simulink library "Control_lib"  (Simulink 7.4)
settings: Solver=ode45  StartTime=0.0  StopTime=10.0  RelTol=1e-3
values from neighbouring files (symbols this model uses):
  f1 = (I_y-I_z)/I_x    [quadrocopter_param.m]
  f2 = rot.J_z/I_x    [quadrocopter_param.m]
  f3 = (I_z-I_x)/I_y    [quadrocopter_param.m]
  f4 = rot.J_z/I_y    [quadrocopter_param.m]
  f5 = (I_x-I_y)/I_z    [quadrocopter_param.m]
  g = 9.81    [quadrocopter_param.m]
  I_x = elec.I_x+bat.I_x+2*boom.I_1x+2*boom.I_1y+2*mot.I_1x+2*mot.I_1y+                             2*rot.I_1x+2*rot.I_1y    [quadrocopter_param.m]
  I_y = elec.I_y+bat.I_y+2*boom.I_1x+2*boom.I_1y+2*mot.I_1x+2*mot.I_1y+                             2*rot.I_1x+2*rot.I_1y    [quadrocopter_param.m]
  I_z = elec.I_z+bat.I_z+4*boom.I_1z+4*mot.I_1z+4*rot.I_1z    [quadrocopter_param.m]
  m = m*1.2    [quadrocopter_param.m]
  phi0 = 0    [quadrocopter_param.m]
  r_phi0 = 0    [quadrocopter_param.m]
  r_psi0 = 0    [quadrocopter_param.m]
  r_theta0 = 0    [quadrocopter_param.m]
  theta0 = 0    [quadrocopter_param.m]
  Ts = 0.005    [quadrocopter_param.m]
undefined symbols (not defined in the file or in its folder): boom, DiscIntNeverNeededParam
libraries: Copter_Library x10, simulink x5
settings Model: Creator=roczit00  LastModifiedBy=robert

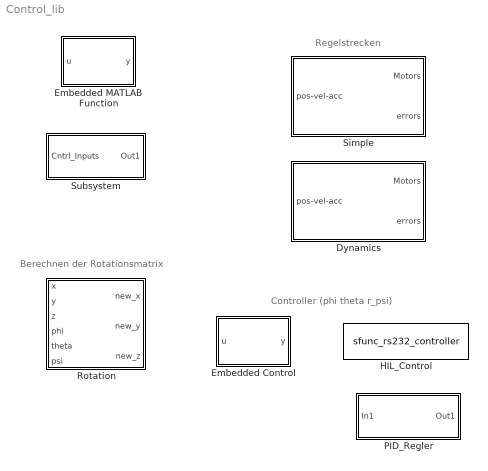
== system Control_lib ==
  note: Regelstrecken
  note: Berechnen der Rotationsmatrix
  note: Controller (phi theta r_psi)
  Dynamics : Subsystem
  Embedded Control : Stateflow chart
  Embedded MATLAB Function : Stateflow chart
  HIL_Control : S-Function  FunctionName=sfunc_rs232_controller  Parameters=Config  EnableBusSupport=off  mask{enabled=off}
      mask prompts: enabled "Enable this Block:"
      mask init:
      | Config.Enabled = enabled;
  PID_Regler : Subsystem
  Rotation : Subsystem
  Simple : Subsystem
  Subsystem : Subsystem  mask{G=9.81}
      mask prompts: G "Erdbeschleunigung [m/s²]:"
      mask init:
      | g = G;

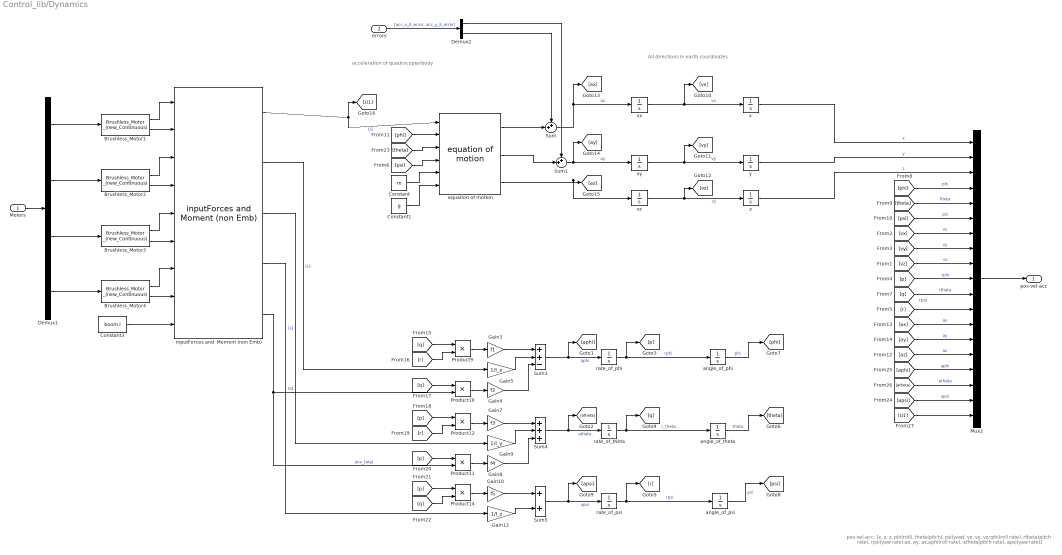
== system Control_lib/Dynamics ==
  note: rpsi
  note: pos-vel-acc: [x, y, z, phi(roll), theta(pitch), psi(yaw), vx, vy, vz,rphi(roll rate), rtheta(pitch rate), rpsi(yaw rate),ax, ay, az,aphi(roll rate), atheta(pitch rate), apsi(yaw rate)]
  note: All directions in earth coordinates
  note: acceleration of quadrocopterbody
  Motors : Inport  OutDataType=fixdt(1, 16)  OutScaling=2^0
  errors : Inport  Port=2  OutDataType=fixdt(1, 16)  OutScaling=2^0
  Brushless_Motor{1..4} (4 alike) : Copter_Library/Brushless_Motor _(new_Continuous)  SystemSampleTime=-1  M_error=0
  Constant : Constant  Value=m  OutDataType=fixdt(1, 16)  OutScaling=2^0
  Constant1 : Constant  Value=g  OutDataType=fixdt(1, 16)  OutScaling=2^0
  Constant3 : Constant  Value=boom.l  OutDataType=fixdt(1, 16)  OutScaling=2^0
  Demux1 : Demux
  Demux2 : Demux  Outputs=2
  Gain10 : Gain  Gain=f5  ParameterDataType=fixdt(1, 16)  ParameterScaling=2^0  OutDataType=fixdt(1, 16)  OutScaling=2^0
  Gain12 : Gain  Gain=1/I_z  ParameterDataType=fixdt(1, 16)  ParameterScaling=2^0  OutDataType=fixdt(1, 16)  OutScaling=2^0
  Gain3 : Gain  Gain=f1  ParameterDataType=fixdt(1, 16)  ParameterScaling=2^0  OutDataType=fixdt(1, 16)  OutScaling=2^0
  Gain4 : Gain  Gain=f2  ParameterDataType=fixdt(1, 16)  ParameterScaling=2^0  OutDataType=fixdt(1, 16)  OutScaling=2^0
  Gain5 : Gain  Gain=1/I_x  ParameterDataType=fixdt(1, 16)  ParameterScaling=2^0  OutDataType=fixdt(1, 16)  OutScaling=2^0
  Gain7 : Gain  Gain=f3  ParameterDataType=fixdt(1, 16)  ParameterScaling=2^0  OutDataType=fixdt(1, 16)  OutScaling=2^0
  Gain8 : Gain  Gain=f4  ParameterDataType=fixdt(1, 16)  ParameterScaling=2^0  OutDataType=fixdt(1, 16)  OutScaling=2^0
  Gain9 : Gain  Gain=1/I_y  ParameterDataType=fixdt(1, 16)  ParameterScaling=2^0  OutDataType=fixdt(1, 16)  OutScaling=2^0
  Mux2 : Mux  Inputs=19
  Product{9..12,14} (5 alike) : Product  OutDataType=fixdt(1, 16)  OutScaling=2^0  RndMeth=Zero
  Sum : Sum  Inputs=++|  OutDataType=fixdt(1, 16)  OutScaling=2^0
  Sum1 : Sum  Inputs=++|  OutDataType=fixdt(1, 16)  OutScaling=2^0
  Sum3 : Sum  Inputs=++-  OutDataType=fixdt(1, 16)  OutScaling=2^0
  Sum4 : Sum  Inputs=+++  OutDataType=fixdt(1, 16)  OutScaling=2^0
  Sum5 : Sum  OutDataType=fixdt(1, 16)  OutScaling=2^0
  angle_of_phi : Integrator  InitialCondition=phi0
  angle_of_psi : Integrator
  angle_of_theta : Integrator  InitialCondition=theta0
  equation of motion : Copter_Library/equation of motion  SystemSampleTime=-1
  inputForces and  Moment (non Emb) : Copter_Library/inputForces and  Moment (non Emb)  SystemSampleTime=-1
  rate_of_phi : Integrator  InitialCondition=r_phi0
  rate_of_psi : Integrator  InitialCondition=r_psi0
  rate_of_theta : Integrator  InitialCondition=r_theta0
  vx : Integrator
  vy : Integrator
  vz : Integrator
  x : Integrator
  y : Integrator
  z : Integrator
  pos-vel-acc : Outport  OutDataType=fixdt(1, 16)  OutScaling=2^0
  wires:
  [apsi] -> Mux2/18  "apsi"
  [atheta] -> Mux2/17  "atheta"
  [aphi] -> Mux2/16  "aphi"
  [az] -> Mux2/15  "az"
  [ay] -> Mux2/14  "ay"
  [ax] -> Mux2/13  "ax"
  [r] -> Mux2/12
  [q] -> Mux2/11  "rtheta"
  [p] -> Mux2/10  "rphi"
  [vz] -> Mux2/9  "vz"
  [vy] -> Mux2/8  "vy"
  [vx] -> Mux2/7  "vx"
  [psi] -> Mux2/6  "psi"
  [theta] -> Mux2/5  "theta"
  [phi] -> Mux2/4  "phi"
  z/1 -> Mux2/3  "z"
  Mux2/1 -> pos-vel-acc/1
  errors/1 -> Demux2/1  "[acc_x_E_error, acc_y_E_error]"
  Motors/1 -> Demux1/1
  Demux1/3 -> Brushless_Motor3/1
  Demux1/4 -> Brushless_Motor4/1
  Demux1/2 -> Brushless_Motor2/1
  Demux1/1 -> Brushless_Motor1/1
  vx/1 -> [vx], x/1  "vx"
  vy/1 -> [vy], y/1  "vy"
  vz/1 -> [vz], z/1  "vz"
  Constant3/1 -> inputForces and  Moment (non Emb)/9
  Sum5/1 -> [apsi], rate_of_psi/1  "apsi"
  inputForces and  Moment (non Emb)/4 -> Gain12/1  "U4"
  Gain12/1 -> Sum5/2
  Gain10/1 -> Sum5/1
  Product14/1 -> Gain10/1
  [q] -> Product14/2
  [p] -> Product14/1
  Sum4/1 -> [atheta], rate_of_theta/1  "atheta"
  inputForces and  Moment (non Emb)/3 -> Gain9/1  "U3"
  Gain8/1 -> Sum4/3
  Gain9/1 -> Sum4/2
  Product11/1 -> Gain8/1
  [p] -> Product11/1
  Gain7/1 -> Sum4/1
  Product12/1 -> Gain7/1
  [r] -> Product12/2
  [p] -> Product12/1
  Sum3/1 -> [aphi], rate_of_phi/1  "aphi"
  Gain4/1 -> Sum3/3
  Gain5/1 -> Sum3/2
  inputForces and  Moment (non Emb)/2 -> Gain5/1  "U2"
  Product10/1 -> Gain4/1
  [q] -> Product10/1
  Gain3/1 -> Sum3/1
  Product9/1 -> Gain3/1
  [r] -> Product9/2
  [q] -> Product9/1
  inputForces and  Moment (non Emb)/5 -> Product11/2, Product10/2  "anv_total"
  angle_of_phi/1 -> [phi]  "phi"
  angle_of_theta/1 -> [theta]  "theta"
  angle_of_psi/1 -> [psi]  "psi"
  rate_of_phi/1 -> [p], angle_of_phi/1  "rphi"
  rate_of_theta/1 -> angle_of_theta/1, [q]  "r_theta"
  rate_of_psi/1 -> angle_of_psi/1, [r]  "rpsi"
  Brushless_Motor1/1 -> inputForces and  Moment (non Emb)/1
  Brushless_Motor1/2 -> inputForces and  Moment (non Emb)/2
  Brushless_Motor2/1 -> inputForces and  Moment (non Emb)/3
  Brushless_Motor2/2 -> inputForces and  Moment (non Emb)/4
  Brushless_Motor3/1 -> inputForces and  Moment (non Emb)/5
  Brushless_Motor3/2 -> inputForces and  Moment (non Emb)/6
  Brushless_Motor4/1 -> inputForces and  Moment (non Emb)/7
  Brushless_Motor4/2 -> inputForces and  Moment (non Emb)/8
  x/1 -> Mux2/1  "x"
  y/1 -> Mux2/2  "y"
  Sum1/1 -> [ay], vy/1  "ay"
  Sum/1 -> [ax], vx/1  "ax"
  Demux2/2 -> Sum/1
  Demux2/1 -> Sum1/1
  equation of motion/3 -> [az], vz/1
  equation of motion/2 -> Sum1/2
  equation of motion/1 -> Sum/2
  inputForces and  Moment (non Emb)/1 -> equation of motion/1, [U1]  "U1"
  [phi] -> equation of motion/2
  [theta] -> equation of motion/3
  [psi] -> equation of motion/4
  Constant/1 -> equation of motion/5
  Constant1/1 -> equation of motion/6
  [U1] -> Mux2/19

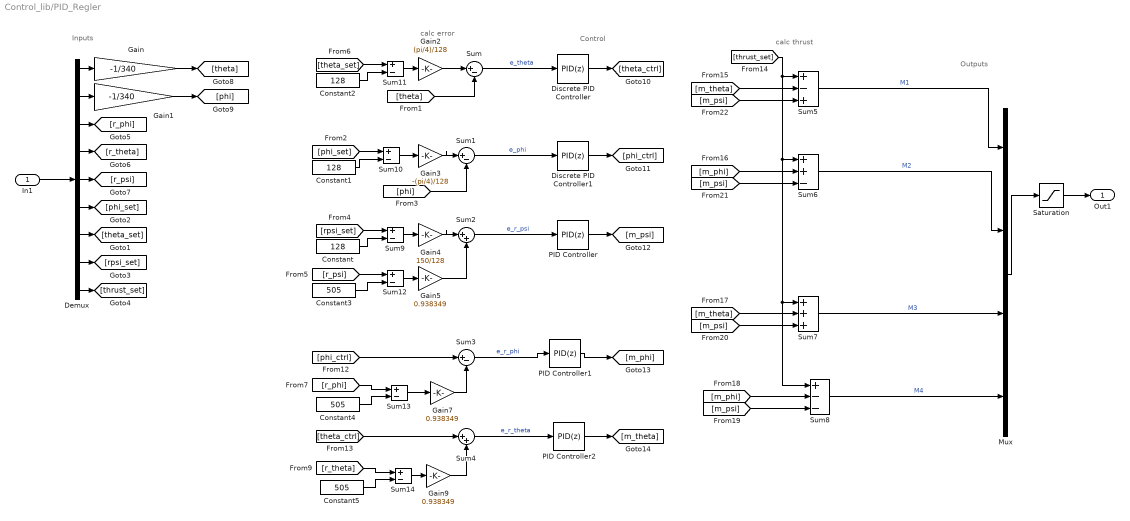
== system Control_lib/PID_Regler ==
  note: Inputs
  note: calc error
  note: Outputs
  note: Control
  note: calc thrust
  In1 : Inport  OutDataType=fixdt(1, 16)  OutScaling=2^0
  Constant : Constant  Value=128  OutDataType=fixdt(1, 16)  OutScaling=2^0
  Constant1 : Constant  Value=128  OutDataType=fixdt(1, 16)  OutScaling=2^0
  Constant2 : Constant  Value=128  OutDataType=fixdt(1, 16)  OutScaling=2^0
  Constant3 : Constant  Value=505  OutDataType=fixdt(1, 16)  OutScaling=2^0
  Constant4 : Constant  Value=505  OutDataType=fixdt(1, 16)  OutScaling=2^0
  Constant5 : Constant  Value=505  OutDataType=fixdt(1, 16)  OutScaling=2^0
  Demux : Demux  Outputs=9
  Discrete PID Controller : simulink/Continuous/PID Controller  DialogController=pidpack.PIDConfig.pidDDGCreate  DialogControllerArgs=DataTag0  SystemSampleTime=-1  Controller=PID  TimeDomain=Discrete-time  SampleTime=Ts  IntegratorMethod=Forward Euler  FilterMethod=Forward Euler  Form=Ideal  P=150  I=0.5  D=0  N=0  InitialConditionSource=internal  InitialConditionForIntegrator=0  InitialConditionForFilter=0  ExternalReset=none  ZeroCross=off  LimitOutput=off  UpperSaturationLimit=inf  LowerSaturationLimit=-inf  LinearizeAsGain=off  AntiWindupMode=none  Kb=1  TrackingMode=off  Kt=1  PParamMin=[]  PParamMax=[]  IParamMin=[]  IParamMax=[]  DParamMin=[]  DParamMax=[]  NParamMin=[]  NParamMax=[]  KbParamMin=[]  KbParamMax=[]  KtParamMin=[]  KtParamMax=[]  POutMin=[]  POutMax=[]  IOutMin=[]  IOutMax=[]  DOutMin=[]  DOutMax=[]  NOutMin=[]  NOutMax=[]  KbOutMin=[]  KbOutMax=[]  KtOutMin=[]  KtOutMax=[]  IntegratorOutMin=[]  IntegratorOutMax=[]  FilterOutMin=[]  FilterOutMax=[]  SumOutMin=[]  SumOutMax=[]  SumI1OutMin=[]  SumI1OutMax=[]  SumI2OutMin=[]  SumI2OutMax=[]  SumI3OutMin=[]  SumI3OutMax=[]  SumDOutMin=[]  SumDOutMax=[]  SaturationOutMin=[]  SaturationOutMax=[]  IntegratorContinuousStateAttributes=''  IntegratorStateMustResolveToSignalObject=off  IntegratorRTWStateStorageClass=Auto  FilterContinuousStateAttributes=''  FilterStateMustResolveToSignalObject=off  FilterRTWStateStorageClass=Auto
  Discrete PID Controller1 : simulink/Continuous/PID Controller  DialogController=pidpack.PIDConfig.pidDDGCreate  DialogControllerArgs=DataTag1  SystemSampleTime=-1  Controller=PID  TimeDomain=Discrete-time  SampleTime=Ts  IntegratorMethod=Forward Euler  FilterMethod=Forward Euler  Form=Ideal  P=150  I=0.5  D=0  N=0  InitialConditionSource=internal  InitialConditionForIntegrator=0  InitialConditionForFilter=0  ExternalReset=none  ZeroCross=off  LimitOutput=off  UpperSaturationLimit=inf  LowerSaturationLimit=-inf  LinearizeAsGain=off  AntiWindupMode=none  Kb=1  TrackingMode=off  Kt=1  PParamMin=[]  PParamMax=[]  IParamMin=[]  IParamMax=[]  DParamMin=[]  DParamMax=[]  NParamMin=[]  NParamMax=[]  KbParamMin=[]  KbParamMax=[]  KtParamMin=[]  KtParamMax=[]  POutMin=[]  POutMax=[]  IOutMin=[]  IOutMax=[]  DOutMin=[]  DOutMax=[]  NOutMin=[]  NOutMax=[]  KbOutMin=[]  KbOutMax=[]  KtOutMin=[]  KtOutMax=[]  IntegratorOutMin=[]  IntegratorOutMax=[]  FilterOutMin=[]  FilterOutMax=[]  SumOutMin=[]  SumOutMax=[]  SumI1OutMin=[]  SumI1OutMax=[]  SumI2OutMin=[]  SumI2OutMax=[]  SumI3OutMin=[]  SumI3OutMax=[]  SumDOutMin=[]  SumDOutMax=[]  SaturationOutMin=[]  SaturationOutMax=[]  IntegratorContinuousStateAttributes=''  IntegratorStateMustResolveToSignalObject=off  IntegratorRTWStateStorageClass=Auto  FilterContinuousStateAttributes=''  FilterStateMustResolveToSignalObject=off  FilterRTWStateStorageClass=Auto
  Gain : Gain  Gain=-1/340  ParameterDataType=fixdt(1, 16)  ParameterScaling=2^0  OutDataType=fixdt(1, 16)  OutScaling=2^0
  Gain1 : Gain  Gain=-1/340  ParameterDataType=fixdt(1, 16)  ParameterScaling=2^0  OutDataType=fixdt(1, 16)  OutScaling=2^0
  Gain2 : Gain  Gain=(pi/4)/128  ParameterDataType=fixdt(1, 16)  ParameterScaling=2^0  OutDataType=fixdt(1, 16)  OutScaling=2^0
  Gain3 : Gain  Gain=-(pi/4)/128  ParameterDataType=fixdt(1, 16)  ParameterScaling=2^0  OutDataType=fixdt(1, 16)  OutScaling=2^0
  Gain4 : Gain  Gain=150/128  ParameterDataType=fixdt(1, 16)  ParameterScaling=2^0  OutDataType=fixdt(1, 16)  OutScaling=2^0
  Gain5 : Gain  Gain=0.938349  ParameterDataType=fixdt(1, 16)  ParameterScaling=2^0  OutDataType=fixdt(1, 16)  OutScaling=2^0
  Gain7 : Gain  Gain=0.938349  ParameterDataType=fixdt(1, 16)  ParameterScaling=2^0  OutDataType=fixdt(1, 16)  OutScaling=2^0
  Gain9 : Gain  Gain=0.938349  ParameterDataType=fixdt(1, 16)  ParameterScaling=2^0  OutDataType=fixdt(1, 16)  OutScaling=2^0
  Mux : Mux
  PID Controller : simulink/Continuous/PID Controller  DialogController=pidpack.PIDConfig.pidDDGCreate  DialogControllerArgs=DataTag2  SystemSampleTime=-1  Controller=PID  TimeDomain=Discrete-time  SampleTime=Ts  IntegratorMethod=Forward Euler  FilterMethod=Forward Euler  Form=Ideal  P=60  I=0.5  D=0  N=0  InitialConditionSource=internal  InitialConditionForIntegrator=0  InitialConditionForFilter=0  ExternalReset=none  ZeroCross=off  LimitOutput=off  UpperSaturationLimit=inf  LowerSaturationLimit=-inf  LinearizeAsGain=off  AntiWindupMode=none  Kb=1  TrackingMode=off  Kt=1  PParamMin=[]  PParamMax=[]  IParamMin=[]  IParamMax=[]  DParamMin=[]  DParamMax=[]  NParamMin=[]  NParamMax=[]  KbParamMin=[]  KbParamMax=[]  KtParamMin=[]  KtParamMax=[]  POutMin=[]  POutMax=[]  IOutMin=[]  IOutMax=[]  DOutMin=[]  DOutMax=[]  NOutMin=[]  NOutMax=[]  KbOutMin=[]  KbOutMax=[]  KtOutMin=[]  KtOutMax=[]  IntegratorOutMin=[]  IntegratorOutMax=[]  FilterOutMin=[]  FilterOutMax=[]  SumOutMin=[]  SumOutMax=[]  SumI1OutMin=[]  SumI1OutMax=[]  SumI2OutMin=[]  SumI2OutMax=[]  SumI3OutMin=[]  SumI3OutMax=[]  SumDOutMin=[]  SumDOutMax=[]  SaturationOutMin=[]  SaturationOutMax=[]  IntegratorContinuousStateAttributes=''  IntegratorStateMustResolveToSignalObject=off  IntegratorRTWStateStorageClass=Auto  FilterContinuousStateAttributes=''  FilterStateMustResolveToSignalObject=off  FilterRTWStateStorageClass=Auto
  PID Controller1 : simulink/Continuous/PID Controller  DialogController=pidpack.PIDConfig.pidDDGCreate  DialogControllerArgs=DataTag3  SystemSampleTime=-1  Controller=PID  TimeDomain=Discrete-time  SampleTime=Ts  IntegratorMethod=Forward Euler  FilterMethod=Forward Euler  Form=Ideal  P=60  I=0.5  D=0  N=0  InitialConditionSource=internal  InitialConditionForIntegrator=0  InitialConditionForFilter=0  ExternalReset=none  ZeroCross=off  LimitOutput=off  UpperSaturationLimit=inf  LowerSaturationLimit=-inf  LinearizeAsGain=off  AntiWindupMode=none  Kb=1  TrackingMode=off  Kt=1  PParamMin=[]  PParamMax=[]  IParamMin=[]  IParamMax=[]  DParamMin=[]  DParamMax=[]  NParamMin=[]  NParamMax=[]  KbParamMin=[]  KbParamMax=[]  KtParamMin=[]  KtParamMax=[]  POutMin=[]  POutMax=[]  IOutMin=[]  IOutMax=[]  DOutMin=[]  DOutMax=[]  NOutMin=[]  NOutMax=[]  KbOutMin=[]  KbOutMax=[]  KtOutMin=[]  KtOutMax=[]  IntegratorOutMin=[]  IntegratorOutMax=[]  FilterOutMin=[]  FilterOutMax=[]  SumOutMin=[]  SumOutMax=[]  SumI1OutMin=[]  SumI1OutMax=[]  SumI2OutMin=[]  SumI2OutMax=[]  SumI3OutMin=[]  SumI3OutMax=[]  SumDOutMin=[]  SumDOutMax=[]  SaturationOutMin=[]  SaturationOutMax=[]  IntegratorContinuousStateAttributes=''  IntegratorStateMustResolveToSignalObject=off  IntegratorRTWStateStorageClass=Auto  FilterContinuousStateAttributes=''  FilterStateMustResolveToSignalObject=off  FilterRTWStateStorageClass=Auto
  PID Controller2 : simulink/Continuous/PID Controller  DialogController=pidpack.PIDConfig.pidDDGCreate  DialogControllerArgs=DataTag4  SystemSampleTime=-1  Controller=PID  TimeDomain=Discrete-time  SampleTime=Ts  IntegratorMethod=Forward Euler  FilterMethod=Forward Euler  Form=Ideal  P=60  I=0.5  D=0  N=0  InitialConditionSource=internal  InitialConditionForIntegrator=0  InitialConditionForFilter=0  ExternalReset=none  ZeroCross=off  LimitOutput=off  UpperSaturationLimit=inf  LowerSaturationLimit=-inf  LinearizeAsGain=off  AntiWindupMode=none  Kb=1  TrackingMode=off  Kt=1  PParamMin=[]  PParamMax=[]  IParamMin=[]  IParamMax=[]  DParamMin=[]  DParamMax=[]  NParamMin=[]  NParamMax=[]  KbParamMin=[]  KbParamMax=[]  KtParamMin=[]  KtParamMax=[]  POutMin=[]  POutMax=[]  IOutMin=[]  IOutMax=[]  DOutMin=[]  DOutMax=[]  NOutMin=[]  NOutMax=[]  KbOutMin=[]  KbOutMax=[]  KtOutMin=[]  KtOutMax=[]  IntegratorOutMin=[]  IntegratorOutMax=[]  FilterOutMin=[]  FilterOutMax=[]  SumOutMin=[]  SumOutMax=[]  SumI1OutMin=[]  SumI1OutMax=[]  SumI2OutMin=[]  SumI2OutMax=[]  SumI3OutMin=[]  SumI3OutMax=[]  SumDOutMin=[]  SumDOutMax=[]  SaturationOutMin=[]  SaturationOutMax=[]  IntegratorContinuousStateAttributes=''  IntegratorStateMustResolveToSignalObject=off  IntegratorRTWStateStorageClass=Auto  FilterContinuousStateAttributes=''  FilterStateMustResolveToSignalObject=off  FilterRTWStateStorageClass=Auto
  Saturation : Saturate  UpperLimit=255  LowerLimit=0  OutDataType=fixdt(1, 16)  OutScaling=2^0
  Sum : Sum  Inputs=|+-  OutDataType=fixdt(1, 16)  OutScaling=2^0
  Sum1 : Sum  Inputs=|+-  OutDataType=fixdt(1, 16)  OutScaling=2^0
  Sum{9..14} (6 alike) : Sum  Inputs=+-  OutDataType=fixdt(1, 16)  OutScaling=2^0
  Sum2 : Sum  Inputs=|++  OutDataType=fixdt(1, 16)  OutScaling=2^0
  Sum3 : Sum  Inputs=|+-  OutDataType=fixdt(1, 16)  OutScaling=2^0
  Sum4 : Sum  Inputs=|++  OutDataType=fixdt(1, 16)  OutScaling=2^0
  Sum5 : Sum  Inputs=+-+  OutDataType=fixdt(1, 16)  OutScaling=2^0
  Sum6 : Sum  Inputs=++-  OutDataType=fixdt(1, 16)  OutScaling=2^0
  Sum7 : Sum  Inputs=+++  OutDataType=fixdt(1, 16)  OutScaling=2^0
  Sum8 : Sum  Inputs=+--  OutDataType=fixdt(1, 16)  OutScaling=2^0
  Out1 : Outport  OutDataType=fixdt(1, 16)  OutScaling=2^0
  wires:
  In1/1 -> Demux/1
  Demux/2 -> Gain1/1
  Demux/1 -> Gain/1
  Demux/3 -> [r_phi]
  Demux/4 -> [r_theta]
  Demux/5 -> [r_psi]
  Demux/6 -> [phi_set]
  Demux/7 -> [theta_set]
  Demux/8 -> [rpsi_set]
  Demux/9 -> [thrust_set]
  Gain/1 -> [theta]
  Gain1/1 -> [phi]
  [theta] -> Sum/2
  Sum/1 -> Discrete PID Controller/1  "e_theta"
  [phi] -> Sum1/2
  Sum1/1 -> Discrete PID Controller1/1  "e_phi"
  Sum2/1 -> PID Controller/1  "e_r_psi"
  Sum3/1 -> PID Controller1/1  "e_r_phi"
  Sum4/1 -> PID Controller2/1  "e_r_theta"
  Sum5/1 -> Mux/1  "M1"
  Sum8/1 -> Mux/4  "M4"
  Sum7/1 -> Mux/3  "M3"
  Sum6/1 -> Mux/2  "M2"
  Discrete PID Controller1/1 -> [phi_ctrl]
  Discrete PID Controller/1 -> [theta_ctrl]
  PID Controller/1 -> [m_psi]
  PID Controller1/1 -> [m_phi]
  PID Controller2/1 -> [m_theta]
  [thrust_set] -> Sum5/1, Sum6/1, Sum7/1, Sum8/1
  [m_theta] -> Sum5/2
  [m_psi] -> Sum5/3
  [m_phi] -> Sum6/2
  [m_psi] -> Sum6/3
  [m_theta] -> Sum7/2
  [m_psi] -> Sum7/3
  [m_phi] -> Sum8/2
  [m_psi] -> Sum8/3
  Mux/1 -> Saturation/1
  Saturation/1 -> Out1/1
  [rpsi_set] -> Sum9/1
  Constant/1 -> Sum9/2
  [phi_set] -> Sum10/1
  Constant1/1 -> Sum10/2
  [theta_set] -> Sum11/1
  Constant2/1 -> Sum11/2
  [r_psi] -> Sum12/1
  Constant3/1 -> Sum12/2
  Constant4/1 -> Sum13/2
  [r_phi] -> Sum13/1
  Constant5/1 -> Sum14/2
  [r_theta] -> Sum14/1
  Sum10/1 -> Gain3/1
  Sum11/1 -> Gain2/1
  Gain2/1 -> Sum/1
  Gain3/1 -> Sum1/1
  Gain7/1 -> Sum3/2
  Sum13/1 -> Gain7/1
  [theta_ctrl] -> Sum4/1
  Gain9/1 -> Sum4/2
  Sum14/1 -> Gain9/1
  [phi_ctrl] -> Sum3/1
  Sum9/1 -> Gain4/1
  Gain4/1 -> Sum2/1
  Sum12/1 -> Gain5/1
  Gain5/1 -> Sum2/2

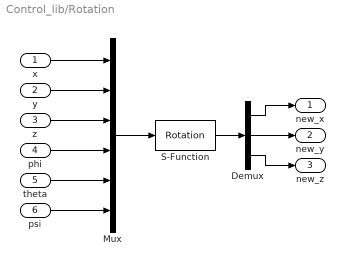
== system Control_lib/Rotation ==
  x : Inport  OutDataType=fixdt(1, 16)  OutScaling=2^0
  y : Inport  Port=2  OutDataType=fixdt(1, 16)  OutScaling=2^0
  z : Inport  Port=3  OutDataType=fixdt(1, 16)  OutScaling=2^0
  phi : Inport  Port=4  OutDataType=fixdt(1, 16)  OutScaling=2^0
  theta : Inport  Port=5  OutDataType=fixdt(1, 16)  OutScaling=2^0
  psi : Inport  Port=6  OutDataType=fixdt(1, 16)  OutScaling=2^0
  Demux : Demux  Outputs=3
  Mux : Mux  Inputs=6
  S-Function : S-Function  FunctionName=Rotation  EnableBusSupport=off
  new_x : Outport  OutDataType=fixdt(1, 16)  OutScaling=2^0
  new_y : Outport  Port=2  OutDataType=fixdt(1, 16)  OutScaling=2^0
  new_z : Outport  Port=3  OutDataType=fixdt(1, 16)  OutScaling=2^0
  wires:
  x/1 -> Mux/1
  y/1 -> Mux/2
  z/1 -> Mux/3
  Mux/1 -> S-Function/1
  S-Function/1 -> Demux/1
  Demux/2 -> new_y/1
  Demux/1 -> new_x/1
  Demux/3 -> new_z/1
  phi/1 -> Mux/4
  theta/1 -> Mux/5
  psi/1 -> Mux/6

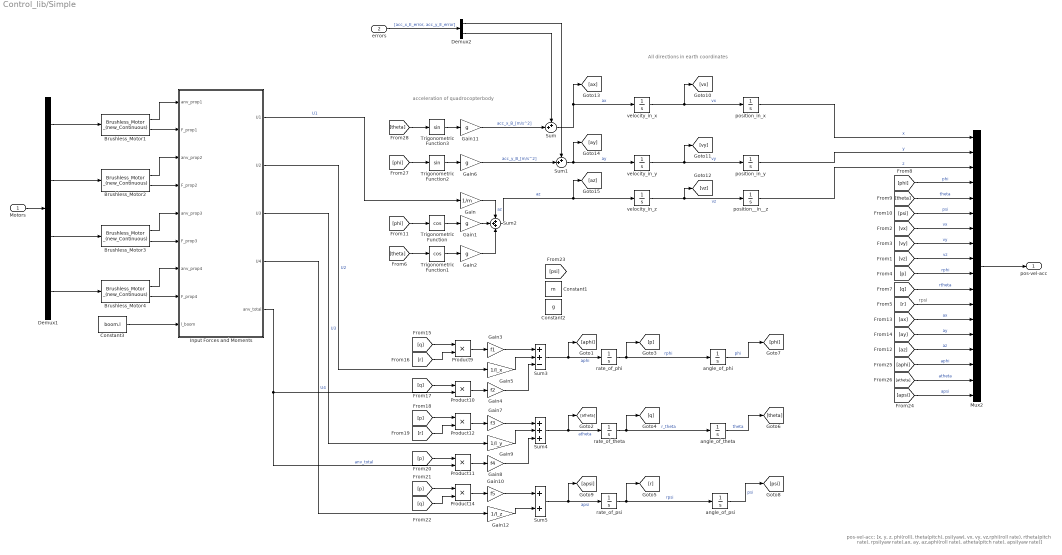
== system Control_lib/Simple ==
  note: acceleration of quadrocopterbody
  note: All directions in earth coordinates
  note: pos-vel-acc: [x, y, z, phi(roll), theta(pitch), psi(yaw), vx, vy, vz,rphi(roll rate), rtheta(pitch rate), rpsi(yaw rate),ax, ay, az,aphi(roll rate), atheta(pitch rate), apsi(yaw rate)]
  note: rpsi
  Motors : Inport  OutDataType=fixdt(1, 16)  OutScaling=2^0
  errors : Inport  Port=2  OutDataType=fixdt(1, 16)  OutScaling=2^0
  Brushless_Motor1 : Copter_Library/Brushless_Motor _(new_Continuous)  SystemSampleTime=-1  M_error=0.1
  Brushless_Motor2 : Copter_Library/Brushless_Motor _(new_Continuous)  SystemSampleTime=-1  M_error=-0.1
  Brushless_Motor3 : Copter_Library/Brushless_Motor _(new_Continuous)  SystemSampleTime=-1  M_error=0.2
  Brushless_Motor4 : Copter_Library/Brushless_Motor _(new_Continuous)  SystemSampleTime=-1  M_error=-0.3
  Constant1 : Constant  Value=m  OutDataType=fixdt(1, 16)  OutScaling=2^0  SampleTime=Ts
  Constant2 : Constant  Value=g  OutDataType=fixdt(1, 16)  OutScaling=2^0  SampleTime=Ts
  Constant3 : Constant  Value=boom.l  OutDataType=fixdt(1, 16)  OutScaling=2^0
  Demux1 : Demux
  Demux2 : Demux  Outputs=2
  Gain : Gain  Gain=1/m  ParameterDataType=fixdt(1, 16)  ParameterScaling=2^0  OutDataType=fixdt(1, 16)  OutScaling=2^0
  Gain{1..2,6,11} (4 alike) : Gain  Gain=g  ParameterDataType=fixdt(1, 16)  ParameterScaling=2^0  OutDataType=fixdt(1, 16)  OutScaling=2^0
  Gain10 : Gain  Gain=f5  ParameterDataType=fixdt(1, 16)  ParameterScaling=2^0  OutDataType=fixdt(1, 16)  OutScaling=2^0
  Gain12 : Gain  Gain=1/I_z  ParameterDataType=fixdt(1, 16)  ParameterScaling=2^0  OutDataType=fixdt(1, 16)  OutScaling=2^0
  Gain3 : Gain  Gain=f1  ParameterDataType=fixdt(1, 16)  ParameterScaling=2^0  OutDataType=fixdt(1, 16)  OutScaling=2^0
  Gain4 : Gain  Gain=f2  ParameterDataType=fixdt(1, 16)  ParameterScaling=2^0  OutDataType=fixdt(1, 16)  OutScaling=2^0
  Gain5 : Gain  Gain=1/I_x  ParameterDataType=fixdt(1, 16)  ParameterScaling=2^0  OutDataType=fixdt(1, 16)  OutScaling=2^0
  Gain7 : Gain  Gain=f3  ParameterDataType=fixdt(1, 16)  ParameterScaling=2^0  OutDataType=fixdt(1, 16)  OutScaling=2^0
  Gain8 : Gain  Gain=f4  ParameterDataType=fixdt(1, 16)  ParameterScaling=2^0  OutDataType=fixdt(1, 16)  OutScaling=2^0
  Gain9 : Gain  Gain=1/I_y  ParameterDataType=fixdt(1, 16)  ParameterScaling=2^0  OutDataType=fixdt(1, 16)  OutScaling=2^0
  Input Forces and Moments : Stateflow chart
  Mux2 : Mux  Inputs=18
  Product{9..12,14} (5 alike) : Product  OutDataType=fixdt(1, 16)  OutScaling=2^0  RndMeth=Zero
  Sum : Sum  Inputs=++|  OutDataType=fixdt(1, 16)  OutScaling=2^0
  Sum1 : Sum  Inputs=++|  OutDataType=fixdt(1, 16)  OutScaling=2^0
  Sum2 : Sum  Inputs=+++  OutDataType=fixdt(1, 16)  OutScaling=2^0
  Sum3 : Sum  Inputs=++-  OutDataType=fixdt(1, 16)  OutScaling=2^0
  Sum4 : Sum  Inputs=+++  OutDataType=fixdt(1, 16)  OutScaling=2^0
  Sum5 : Sum  OutDataType=fixdt(1, 16)  OutScaling=2^0
  Trigonometric Function : Trigonometry  Operator=cos
  Trigonometric Function1 : Trigonometry  Operator=cos
  Trigonometric Function2 : Trigonometry
  Trigonometric Function3 : Trigonometry
  angle_of_phi : Integrator  InitialCondition=phi0
  angle_of_psi : Integrator
  angle_of_theta : Integrator  InitialCondition=theta0
  position__in__z : Integrator
  position_in_x : Integrator
  position_in_y : Integrator
  rate_of_phi : Integrator  InitialCondition=r_phi0
  rate_of_psi : Integrator  InitialCondition=r_psi0
  rate_of_theta : Integrator  InitialCondition=r_theta0
  velocity_in_x : Integrator
  velocity_in_y : Integrator
  velocity_in_z : Integrator
  pos-vel-acc : Outport  OutDataType=fixdt(1, 16)  OutScaling=2^0
  wires:
  Trigonometric Function3/1 -> Gain11/1
  [theta] -> Trigonometric Function3/1
  Trigonometric Function2/1 -> Gain6/1
  [phi] -> Trigonometric Function2/1
  Trigonometric Function1/1 -> Gain2/1
  Trigonometric Function/1 -> Gain1/1
  [theta] -> Trigonometric Function1/1
  [phi] -> Trigonometric Function/1
  Gain2/1 -> Sum2/3
  Gain1/1 -> Sum2/2
  Gain/1 -> Sum2/1  "az"
  Demux2/1 -> Sum1/1
  Demux2/2 -> Sum/1
  Sum/1 -> velocity_in_x/1, [ax]  "ax"
  Gain11/1 -> Sum/2  "acc_x_B_[m/s^2]"
  Gain6/1 -> Sum1/2  "acc_y_B_[m/s^2]"
  Sum1/1 -> velocity_in_y/1, [ay]  "ay"
  position_in_y/1 -> Mux2/2  "y"
  position_in_x/1 -> Mux2/1  "x"
  Sum2/1 -> velocity_in_z/1, [az]  "az"
  Brushless_Motor4/2 -> Input Forces and Moments/8(F_prop4)
  Brushless_Motor4/1 -> Input Forces and Moments/7(anv_prop4)
  Brushless_Motor3/2 -> Input Forces and Moments/6(F_prop3)
  Brushless_Motor3/1 -> Input Forces and Moments/5(anv_prop3)
  Brushless_Motor2/2 -> Input Forces and Moments/4(F_prop2)
  Brushless_Motor2/1 -> Input Forces and Moments/3(anv_prop2)
  Brushless_Motor1/2 -> Input Forces and Moments/2(F_prop1)
  Brushless_Motor1/1 -> Input Forces and Moments/1(anv_prop1)
  rate_of_psi/1 -> [r], angle_of_psi/1  "rpsi"
  rate_of_theta/1 -> [q], angle_of_theta/1  "r_theta"
  rate_of_phi/1 -> angle_of_phi/1, [p]  "rphi"
  angle_of_psi/1 -> [psi]  "psi"
  angle_of_theta/1 -> [theta]  "theta"
  angle_of_phi/1 -> [phi]  "phi"
  Input Forces and Moments/5(anv_total) -> Product10/2, Product11/2  "anv_total"
  [q] -> Product9/1
  [r] -> Product9/2
  Product9/1 -> Gain3/1
  Gain3/1 -> Sum3/1
  [q] -> Product10/1
  Product10/1 -> Gain4/1
  Input Forces and Moments/2(U2) -> Gain5/1  "U2"
  Gain5/1 -> Sum3/2
  Gain4/1 -> Sum3/3
  Sum3/1 -> rate_of_phi/1, [aphi]  "aphi"
  Input Forces and Moments/1(U1) -> Gain/1  "U1"
  [p] -> Product12/1
  [r] -> Product12/2
  Product12/1 -> Gain7/1
  Gain7/1 -> Sum4/1
  [p] -> Product11/1
  Product11/1 -> Gain8/1
  Gain9/1 -> Sum4/2
  Gain8/1 -> Sum4/3
  Input Forces and Moments/3(U3) -> Gain9/1  "U3"
  Sum4/1 -> rate_of_theta/1, [atheta]  "atheta"
  [p] -> Product14/1
  [q] -> Product14/2
  Product14/1 -> Gain10/1
  Gain10/1 -> Sum5/1
  Gain12/1 -> Sum5/2
  Input Forces and Moments/4(U4) -> Gain12/1  "U4"
  Sum5/1 -> rate_of_psi/1, [apsi]  "apsi"
  Constant3/1 -> Input Forces and Moments/9(l_boom)
  velocity_in_z/1 -> position__in__z/1, [vz]  "vz"
  velocity_in_y/1 -> position_in_y/1, [vy]  "vy"
  velocity_in_x/1 -> position_in_x/1, [vx]  "vx"
  Demux1/1 -> Brushless_Motor1/1
  Demux1/2 -> Brushless_Motor2/1
  Demux1/4 -> Brushless_Motor4/1
  Demux1/3 -> Brushless_Motor3/1
  Motors/1 -> Demux1/1
  errors/1 -> Demux2/1  "[acc_x_E_error, acc_y_E_error]"
  Mux2/1 -> pos-vel-acc/1
  position__in__z/1 -> Mux2/3  "z"
  [phi] -> Mux2/4  "phi"
  [theta] -> Mux2/5  "theta"
  [psi] -> Mux2/6  "psi"
  [vx] -> Mux2/7  "vx"
  [vy] -> Mux2/8  "vy"
  [vz] -> Mux2/9  "vz"
  [p] -> Mux2/10  "rphi"
  [q] -> Mux2/11  "rtheta"
  [r] -> Mux2/12
  [ax] -> Mux2/13  "ax"
  [ay] -> Mux2/14  "ay"
  [az] -> Mux2/15  "az"
  [aphi] -> Mux2/16  "aphi"
  [atheta] -> Mux2/17  "atheta"
  [apsi] -> Mux2/18  "apsi"

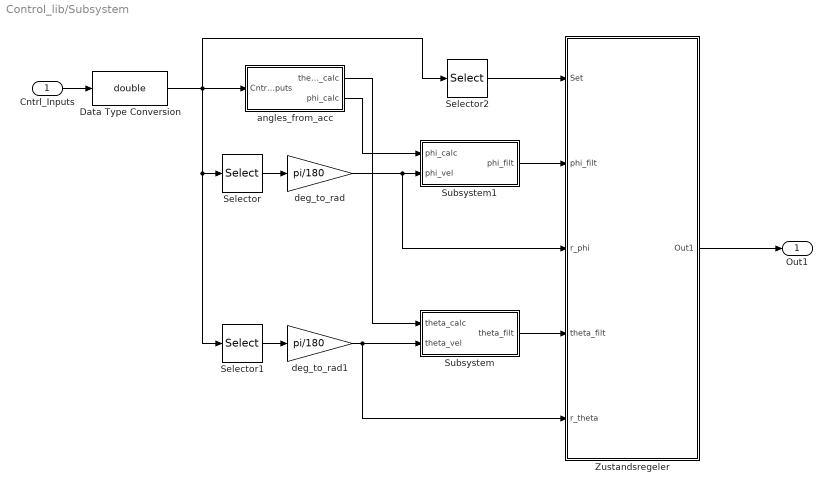
== system Control_lib/Subsystem ==
  Cntrl_Inputs : Inport  OutDataType=fixdt(1, 16)  OutScaling=2^0
  Data Type Conversion : DataTypeConversion  OutDataTypeMode=double  OutDataType=fixdt(1, 16)  OutScaling=2^0  OutDataTypeStr=double
  Selector : Selector  InputPortWidth=12  IndexOptions=Index vector (dialog)  Indices=[8]  OutputSizes=1
  Selector1 : Selector  InputPortWidth=12  IndexOptions=Index vector (dialog)  Indices=[9]  OutputSizes=1
  Selector2 : Selector  InputPortWidth=12  IndexOptions=Index vector (dialog)  Indices=[1 2 3 4]  OutputSizes=1
  Subsystem : Subsystem
  Subsystem1 : Subsystem
  Zustandsregeler : Subsystem  mask{FB_phi=-10, FB_r_phi=-10, FB_theta=-10, FB_r_theta=-10}
      mask prompts: FB_phi "Feedbackfactor phi:"; FB_r_phi "Feedbackfactor r_phi:"; FB_theta "Feedbackfactor theta:"; FB_r_theta "Feedbackfactor theta:"
  angles_from_acc : Subsystem  mask{g=g}
      mask prompts: g "Erdbeschleunigung [m/s²]:"
  deg_to_rad : Gain  Gain=pi/180  ParameterDataType=fixdt(1, 16)  ParameterScaling=2^0  OutDataType=fixdt(1, 16)  OutScaling=2^0  SampleTime=10
  deg_to_rad1 : Gain  Gain=pi/180  ParameterDataType=fixdt(1, 16)  ParameterScaling=2^0  OutDataType=fixdt(1, 16)  OutScaling=2^0  SampleTime=10
  Out1 : Outport  OutDataType=fixdt(1, 16)  OutScaling=2^0
  wires:
  angles_from_acc/2(phi_calc) -> Subsystem1/1(phi_calc)
  angles_from_acc/1(theta_calc) -> Subsystem/1(theta_calc)
  Selector2/1 -> Zustandsregeler/1(Set)
  Cntrl_Inputs/1 -> Data Type Conversion/1
  Data Type Conversion/1 -> angles_from_acc/1(Cntrl_Inputs), Selector2/1, Selector/1, Selector1/1
  Selector/1 -> deg_to_rad/1
  deg_to_rad/1 -> Subsystem1/2(phi_vel), Zustandsregeler/3(r_phi)
  Selector1/1 -> deg_to_rad1/1
  deg_to_rad1/1 -> Subsystem/2(theta_vel), Zustandsregeler/5(r_theta)
  Zustandsregeler/1(Out1) -> Out1/1
  Subsystem1/1(phi_filt) -> Zustandsregeler/2(phi_filt)
  Subsystem/1(theta_filt) -> Zustandsregeler/4(theta_filt)

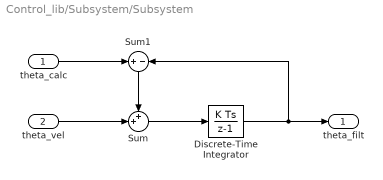
== system Control_lib/Subsystem/Subsystem ==
  theta_calc : Inport  OutDataType=fixdt(1, 16)  OutScaling=2^0
  theta_vel : Inport  Port=2  OutDataType=fixdt(1, 16)  OutScaling=2^0
  Discrete-Time Integrator : DiscreteIntegrator  InitialCondition=theta0  SampleTime=Ts  OutDataType=fixdt(1, 16)  OutScaling=2^0  ICPrevOutput=DiscIntNeverNeededParam  ICPrevScaledInput=DiscIntNeverNeededParam
  Sum : Sum  Inputs=++|  OutDataType=fixdt(1, 16)  OutScaling=2^0
  Sum1 : Sum  Inputs=+|-  OutDataType=fixdt(1, 16)  OutScaling=2^0
  theta_filt : Outport  OutDataType=fixdt(1, 16)  OutScaling=2^0
  wires:
  Discrete-Time Integrator/1 -> theta_filt/1, Sum1/2
  Sum/1 -> Discrete-Time Integrator/1
  theta_vel/1 -> Sum/2
  Sum1/1 -> Sum/1
  theta_calc/1 -> Sum1/1

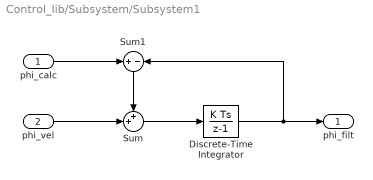
== system Control_lib/Subsystem/Subsystem1 ==
  phi_calc : Inport  OutDataType=fixdt(1, 16)  OutScaling=2^0
  phi_vel : Inport  Port=2  OutDataType=fixdt(1, 16)  OutScaling=2^0
  Discrete-Time Integrator : DiscreteIntegrator  InitialCondition=theta0  SampleTime=Ts  OutDataType=fixdt(1, 16)  OutScaling=2^0  ICPrevOutput=DiscIntNeverNeededParam  ICPrevScaledInput=DiscIntNeverNeededParam
  Sum : Sum  Inputs=++|  OutDataType=fixdt(1, 16)  OutScaling=2^0
  Sum1 : Sum  Inputs=+|-  OutDataType=fixdt(1, 16)  OutScaling=2^0
  phi_filt : Outport  OutDataType=fixdt(1, 16)  OutScaling=2^0
  wires:
  Discrete-Time Integrator/1 -> phi_filt/1, Sum1/2
  Sum/1 -> Discrete-Time Integrator/1
  phi_vel/1 -> Sum/2
  Sum1/1 -> Sum/1
  phi_calc/1 -> Sum1/1

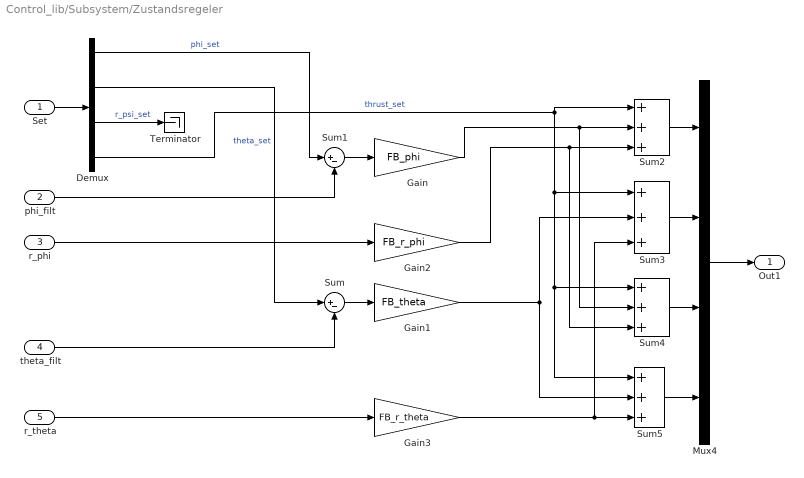
== system Control_lib/Subsystem/Zustandsregeler ==
  Set : Inport  OutDataType=fixdt(1, 16)  OutScaling=2^0
  phi_filt : Inport  Port=2  OutDataType=fixdt(1, 16)  OutScaling=2^0
  r_phi : Inport  Port=3  OutDataType=fixdt(1, 16)  OutScaling=2^0
  theta_filt : Inport  Port=4  OutDataType=fixdt(1, 16)  OutScaling=2^0
  r_theta : Inport  Port=5  OutDataType=fixdt(1, 16)  OutScaling=2^0
  Demux : Demux
  Gain : Gain  Gain=FB_phi  ParameterDataType=fixdt(1, 16)  ParameterScaling=2^0  OutDataType=fixdt(1, 16)  OutScaling=2^0
  Gain1 : Gain  Gain=FB_theta  ParameterDataType=fixdt(1, 16)  ParameterScaling=2^0  OutDataType=fixdt(1, 16)  OutScaling=2^0
  Gain2 : Gain  Gain=FB_r_phi  ParameterDataType=fixdt(1, 16)  ParameterScaling=2^0  OutDataType=fixdt(1, 16)  OutScaling=2^0
  Gain3 : Gain  Gain=FB_r_theta  ParameterDataType=fixdt(1, 16)  ParameterScaling=2^0  OutDataType=fixdt(1, 16)  OutScaling=2^0
  Mux4 : Mux
  Sum : Sum  Inputs=|+-  OutDataType=fixdt(1, 16)  OutScaling=2^0
  Sum1 : Sum  Inputs=|+-  OutDataType=fixdt(1, 16)  OutScaling=2^0
  Sum{2..5} (4 alike) : Sum  Inputs=+++  OutDataType=fixdt(1, 16)  OutScaling=2^0
  Terminator : Terminator
  Out1 : Outport  OutDataType=fixdt(1, 16)  OutScaling=2^0
  wires:
  Mux4/1 -> Out1/1
  Sum2/1 -> Mux4/1
  Sum3/1 -> Mux4/2
  Sum4/1 -> Mux4/3
  Sum5/1 -> Mux4/4
  Sum1/1 -> Gain/1
  Gain/1 -> Sum2/2, Sum4/2
  Gain1/1 -> Sum5/2, Sum3/2
  Sum/1 -> Gain1/1
  Gain2/1 -> Sum2/3, Sum4/3
  Gain3/1 -> Sum5/3, Sum3/3
  Set/1 -> Demux/1
  Demux/1 -> Sum1/1  "phi_set"
  Demux/2 -> Sum/1  "theta_set"
  phi_filt/1 -> Sum1/2
  r_phi/1 -> Gain2/1
  theta_filt/1 -> Sum/2
  r_theta/1 -> Gain3/1
  Demux/3 -> Terminator/1  "r_psi_set"
  Demux/4 -> Sum2/1, Sum4/1, Sum5/1, Sum3/1  "thrust_set"

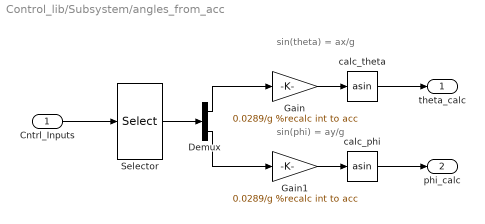
== system Control_lib/Subsystem/angles_from_acc ==
  note: sin(phi) = ay/g
  note: sin(theta) = ax/g
  Cntrl_Inputs : Inport  OutDataType=fixdt(1, 16)  OutScaling=2^0
  Demux : Demux  Outputs=2
  Gain : Gain  Gain=0.0289/g %recalc int to acc  ParameterDataType=fixdt(1, 16)  ParameterScaling=2^0  OutDataType=fixdt(1, 16)  OutScaling=2^0
  Gain1 : Gain  Gain=0.0289/g %recalc int to acc  ParameterDataType=fixdt(1, 16)  ParameterScaling=2^0  OutDataType=fixdt(1, 16)  OutScaling=2^0
  Selector : Selector  InputPortWidth=12  IndexOptions=Index vector (dialog)  Indices=[5 6 ]  OutputSizes=1
  calc_phi : Trigonometry  Operator=asin
  calc_theta : Trigonometry  Operator=asin
  theta_calc : Outport  OutDataType=fixdt(1, 16)  OutScaling=2^0
  phi_calc : Outport  Port=2  OutDataType=fixdt(1, 16)  OutScaling=2^0
  wires:
  Cntrl_Inputs/1 -> Selector/1
  Selector/1 -> Demux/1
  calc_theta/1 -> theta_calc/1
  calc_phi/1 -> phi_calc/1
  Demux/1 -> Gain/1
  Gain/1 -> calc_theta/1
  Demux/2 -> Gain1/1
  Gain1/1 -> calc_phi/1

== matlab function Simple/Input Forces and Moments ==
  data: anv_prop1 input double; F_prop1 input double; anv_prop2 input double; F_prop2 input double; anv_prop3 input double; F_prop3 input double; anv_prop4 input double; U1 output double; F_prop4 input double; U2 output double; U3 output double; U4 output double; l_boom input double; anv_total output double
function [U1, U2, U3, U4, anv_total] = input(anv_prop1,F_prop1,anv_prop2,...
    F_prop2,anv_prop3,F_prop3,anv_prop4,F_prop4,l_boom)
%#eml

% Calculating Thrust in z-axis with respect to body fixed coordinate system
U1 = F_prop1 + F_prop2 + F_prop3 + F_prop4;             % [N]

% Calculating Torque around x-axis (Roll) due to Thrust
U2 = l_boom*(-F_prop4+F_prop2);                         % [Nm]

% Calculating Torque around y-axis (Pitch) due to Thrust
U3 = l_boom*(-F_prop1+F_prop3);                         % [Nm]

% Calculating Torque around z-axis (Yaw) due to Thrust
U4 = l_boom*(F_prop1-F_prop2+F_prop3-F_prop4);          % [Nm]

% Overall propeller speed
anv_total = anv_prop1-anv_prop2+anv_prop3-anv_prop4;    % [rad/s]

== matlab function Embedded Control ==
  settings: updateMethod=DISCRETE  sampleTime=0.01
  data: u input double; y output double
function y = fcn(u)
%#eml
persistent phi_filt theta_filt M1_limited M2_limited M3_limited M4_limited angpsi 
%  first time initialization
if isempty(M1_limited) 
    M1_limited=uint8(0);
end
if isempty(M2_limited) 
    M2_limited=uint8(0);
end
if isempty(M3_limited) 
    M3_limited=uint8(0);
end
if isempty(M4_limited) 
    M4_limited=uint8(0);
end
if isempty(angpsi) 
    angpsi=double(0);
end
if isempty(phi_filt) 
    phi_filt=0.15;
end
if isempty(theta_filt) 
    theta_filt=0.15;
end
Ts = 0.01;
G = 9.81;
Gyro_offset = 505;
sensorSensitivityX = 340;
sensorSensitivityY = 340;
sensorSensitivityZ = 340;
copterState.gyroPOffset = 505;
copterState.gyroROffset = 505;
copterState.gyroYOffset = 505;
% copy inputs to variables with easy to know names
copterState.angVelRRaw =  u(3);
copterState.accYRaw = u(2);
copterState.angVelPRaw = u(4);
copterState.accXRaw = u(1);
copterState.accZRaw = 0; %not available
copterState.angVelYRaw = u(5);
copterState.remoteForceRaw = u(9);
copterState.remotePitchRaw = u(7);
copterState.remoteRollRaw = u(6);
copterState.remoteYawRaw = u(8);
copterState.accY = int16(0);
copterState.accX = int16(0);
copterState.accZ = int16(0);
copterState.angP = int16(0);
copterState.angR = int16(0);
copterState.angVelP = int16(0);
copterState.angVelR = int16(0);
copterState.angVelY = int16(0);
copterState.remotePitch = int16(0);
copterState.remoteRoll = int16(0);
copterState.remoteForce = int16(0);
copterState.remoteYaw = int16(0);
angP = double(0);
angR = double(0);


% Convert Data like in the copter
% Accelerometer
%%%%%%%%%%%%%%%%%
  %/* calculate the physical acceleration values in [(10 * m)/(s^2)], as needed by the control algorithm */
  copterState.accY = int16(((int32(copterState.accYRaw) * G) / sensorSensitivityY) / 10);
  copterState.accX = -int16(((int32(copterState.accXRaw) * G) / sensorSensitivityX) / 10);
  copterState.accZ = -int16(((int32(copterState.accZRaw) * G) / sensorSensitivityZ) / 10);
  %// [ 10000*rad ]
  copterState.angP = -int16(int32(copterState.accXRaw)*1000/340);
  copterState.angR = -int16(int32(copterState.accYRaw)*1000/340);
  
  % Gyroscopes
  %%%%%%%%%%%%%%
   copterState.angVelP     = -int16(double(copterState.angVelPRaw-copterState.gyroPOffset) * 0.938349);
   copterState.angVelR     = int16(double(copterState.angVelRRaw-copterState.gyroROffset) * 0.938349);
   copterState.angVelY     = -int16(double(copterState.angVelYRaw-copterState.gyroYOffset) * 0.938349);
   
   % Remote
   %%%%%%%%%%%%%
  copterState.remotePitch    = int16(0); %//(int16)(maxPitchAngle*(int32)(copterState->remotePitchRaw-128)/maxRemotePitch);
  copterState.remoteRoll     = int16(0); %//(int16)(maxRollAngle*(int32)(copterState->remoteRollRaw-128)/maxRemoteRoll);
  copterState.remoteForce    = int16(copterState.remoteForceRaw); 
  copterState.remoteYaw      = int16(0); %//(int16)(maxYawRate*(int32)(copterState->remoteYawRaw-128)/maxRemoteYaw);

% Set outputs to Values calculated last sample time
y = double([M1_limited;M2_limited;M3_limited;M4_limited]);


   angP = double(copterState.angP)/1000;
   angR = double(copterState.angR)/1000;
   
   %// Filter            ???? 
   %/*angP = angP-angPold*0.63+angPold;
   %angPold = angP;
   %angR = angR-angRold*0.63+angRold;
   %angRold = angR;*/
   angpsi = Ts*double(copterState.angVelY)/100+angpsi;
   
   
    %// Calculate trust modification for the 3 angles
    e_phi=-double(copterState.angVelR)/100 * 41+(double(copterState.remoteRoll)/100-angR) * 34.9;
    e_theta=-double(copterState.angVelP)/100 * 41+(double(copterState.remotePitch)/100-angP) * 34.9;
    e_psi=(double(copterState.remoteYaw)/100-double(copterState.angVelY/100))*20.5- angpsi * 2;

    %//Calculate new setpoints of all motors
    M1 = (copterState.remoteForce-e_theta+e_psi);
    M2 = (copterState.remoteForce+e_phi-e_psi);
    M3 = (copterState.remoteForce+e_theta+e_psi);
    M4 = (copterState.remoteForce-e_phi-e_psi);
    
    %// saturate setpoint of motor1 to 0 if less and 255 if above
    if M1 < 0
      M1_limited = uint8(0);
    else
        if M1 > 255
            M1_limited = uint8(255); 
        else
            M1_limited=uint8(M1);
        end
    end
    
    %// saturate setpoint of motor2 to 0 if less and 255 if above
    if M2 < 0
      M2_limited = uint8(0);
    else
        if M2 > 255
          M2_limited = uint8(255); 
        else
          M2_limited=uint8(M2);
        end
    end

    %// saturate setpoint of motor3 to 0 if less and 255 if above
  if M3 < 0
      M3_limited = uint8(0);
  else
      if M3 > 255
        M3_limited = uint8(255); 
      else
         M3_limited=uint8(M3);
      end
  end
    
    %// saturate setpoint of motor4 to 0 if less and 255 if above
    if M4 < 0
      M4_limited = uint8(0);
    else
        if M4 > 255
           M4_limited = uint8(255); 
        else
           M4_limited=uint8(M4);
        end
    end

== matlab function Embedded MATLAB Function ==
  data: u input double; y output double
function y = fcn(u)
persistent theta_filt_old phi_filt_old;
%#eml
% u = [phi_set, theta_set,rpsi_set, thrust_set, ax_actual, ay__actual, ...
%      az_actual, rphi_actual, rtheta_actual, rpsi_actual]
phi_set       = u(1); % rad
theta_set     = u(2); % rad
r_psi_set      = u(3); % rad/s
thrust_set    = u(4);
ax_actual     = u(5);
ay_actual     = u(6);
az_actual     = u(7);
r_phi_actual   = u(8); % °/s
r_theta_actual = u(9); % °/s
r_psi_actual   = u(10);% °/s
phi0          = u(11);% rad/s
theta0        = u(12);% rad/s

% feedback filter constant
B_theta    = 0.1;
B_phi      = 0.1;
% feedback control
FB_r_phi    = 10;
FB_phi     = 10;
FB_r_theta  = 10;
FB_theta   = 10;
% sample time ==> defined externaly
Ts        = 0.01;

% Static variable created and initialized

if isempty(theta_filt_old) 
    theta_filt_old = double(theta0);
    theta_filt_old = theta_filt_old/1000;
end
if isempty(phi_filt_old) 
    phi_filt_old = double(phi0);
    phi_filt_old = phi_filt_old/1000;
end


%Calculate angles from accelerations
if az_actual ~= 0
    phi = tan(double(ay_actual)/double(az_actual));
    theta = tan(double(-ax_actual)/double(az_actual)); %%% -ax zur korrektur des falschen winkels
else
    % case no working acceleration on x-direction
    if ay_actual < 0
        phi = pi/2;
    else
        phi = -pi/2;
    end
    if ax_actual < 0
        theta = pi/2;
    else
        theta = -pi/2;
    end
end

% Calculate angles from rates
theta_filt = Ts*(double(r_theta_actual)*pi/180 + (theta - theta_filt_old)*B_theta)+theta_filt_old;
phi_filt = Ts*(double(r_phi_actual)*pi/180 + (phi - phi_filt_old)*B_phi)+phi_filt_old;

% copy new values for next run
phi_filt_old   = phi_filt;
theta_filt_old = theta_filt;

% Control
phi_e = double(phi_set) - double(r_phi_actual*pi/180)*FB_r_phi - double(phi_filt)*FB_phi;
theta_e = double(theta_set) - double(r_theta_actual*pi/180)*FB_r_theta - double(theta_filt)*FB_theta;
r_psi_e = double(r_psi_set) - double(r_psi_actual*pi/180);

y = [0; 0; 0; 0];
% calculate trust of Motor 1
y(1) = double(thrust_set/4 + theta_e - r_psi_e); % vorzeichen gedreht
% calculate trust of Motor 2
y(2) = double(thrust_set/4 - phi_e + r_psi_e);
% calculate trust of Motor 3
y(3) = double(thrust_set/4 - theta_e - r_psi_e);
% calculate trust of Motor 4
y(4) = double(thrust_set/4 + phi_e + r_psi_e);
